simulink model "dieu_khien_canh_tay_may"  (R2023b)
settings: Solver=VariableStepAuto  StartTime=0.0  StopTime=3  RelTol=1e-3
values from neighbouring files (symbols this model uses):
  theta1_dot_init = 0    [tinh_toan_canh_tay_may.m]
  theta1_init = 0    [tinh_toan_canh_tay_may.m]
  theta2_dot_init = 0    [tinh_toan_canh_tay_may.m]
  theta2_init = 0    [tinh_toan_canh_tay_may.m]
settings Model: Creator=Admin  LastModifiedBy=Admin

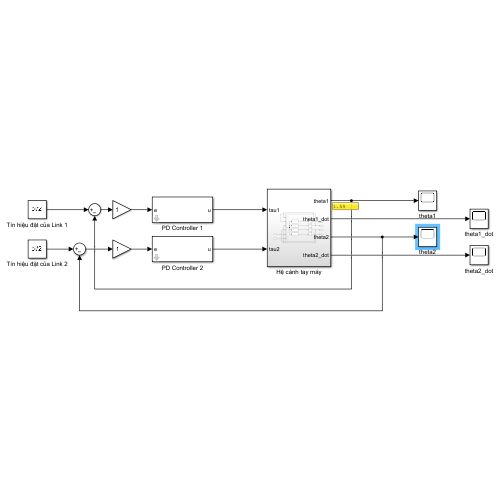
[thumbnail: Simulink's stored preview of the top-level diagram]
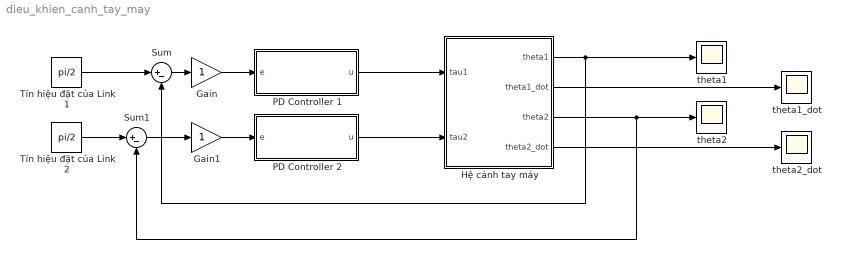
== system dieu_khien_canh_tay_may ==
  Gain : Gain
  Gain1 : Gain
  Hệ cánh tay máy : Subsystem
  PD Controller 1 : Subsystem  mask{Kp1=100, Kd1=20}
      mask prompts: Kp1 "Khâu Tỉ Lệ Kp1"; Kd1 "Khâu Vi Phân Kd1"
  PD Controller 2 : Subsystem  mask{Kp2=100, Kd2=20}
      mask prompts: Kp2 "Khâu Tỉ Lệ Kp2"; Kd2 "Khâu Vi Phân Kd2"
  Sum : Sum  Inputs=|+-
  Sum1 : Sum  Inputs=|+-
  Tín hiệu đặt của Link 1 : Constant  Value=pi/2
  Tín hiệu đặt của Link 2 : Constant  Value=pi/2
  theta1 : Scope
  theta1_dot : Scope
  theta2 : Scope
  theta2_dot : Scope
  wires:
  Hệ cánh tay máy/2(theta1_dot) -> theta1_dot/1
  Hệ cánh tay máy/3(theta2) -> theta2/1, Sum1/2
  Hệ cánh tay máy/4(theta2_dot) -> theta2_dot/1
  PD Controller 2/1(u) -> Hệ cánh tay máy/2(tau2)
  Tín hiệu đặt của Link 2/1 -> Sum1/1
  Tín hiệu đặt của Link 1/1 -> Sum/1
  Sum/1 -> Gain/1
  Sum1/1 -> Gain1/1
  Gain1/1 -> PD Controller 2/1(e)
  Hệ cánh tay máy/1(theta1) -> theta1/1, Sum/2
  Gain/1 -> PD Controller 1/1(e)
  PD Controller 1/1(u) -> Hệ cánh tay máy/1(tau1)

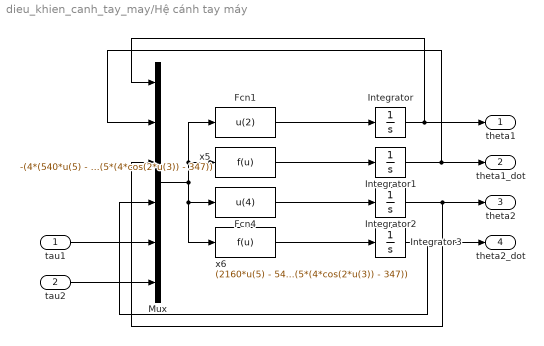
== system dieu_khien_canh_tay_may/Hệ cánh tay máy ==
  tau1 : Inport
  tau2 : Inport  Port=2
  Fcn1 : Fcn  Expr=u(2)
  Fcn4 : Fcn  Expr=u(4)
  Integrator : Integrator  InitialCondition=theta1_init
  Integrator1 : Integrator  InitialCondition=theta1_dot_init
  Integrator2 : Integrator  InitialCondition=theta2_init
  Integrator3 : Integrator  InitialCondition=theta2_dot_init
  Mux : Mux  Inputs=6
  x5 : Fcn  Expr=-(4*(540*u(5) - 540*u(6) + 98*cos(u(1) + 2*u(3)) - 3871*cos(u(1)) + 54*u(2)^2*sin(u(3)) + 54*u(4)^2*sin(u(3)) + 5*u(2)^2*sin(2*u(3)) - 100*u(6)*cos(u(3)) + 108*u(2)*u(4)*sin(u(3))))/(5*(4*cos(2*u(3)) - 347))
  x6 : Fcn  Expr=(2160*u(5) - 5410*u(6) - 1470*cos(u(1) - u(3)) + 392*cos(u(1) + 2*u(3)) + 4900*cos(u(1) + u(3)) - 15484*cos(u(1)) + 541*u(2)^2*sin(u(3)) + 216*u(4)^2*sin(u(3)) + 40*u(2)^2*sin(2*u(3)) + 20*u(4)^2*sin(2*u(3)) + 400*u(5)*cos(u(3)) - 800*u(6)*cos(u(3)) + 432*u(2)*u(4)*sin(u(3)) + 40*u(2)*u(4)*sin(2*u(3)))/(5*(4*cos(2*u(3)) - 347))
  theta1 : Outport
  theta1_dot : Outport  Port=2
  theta2 : Outport  Port=3
  theta2_dot : Outport  Port=4
  wires:
  tau2/1 -> Mux/6
  tau1/1 -> Mux/5
  Integrator1/1 -> Mux/2, theta1_dot/1
  Integrator/1 -> Mux/1, theta1/1
  Integrator2/1 -> Mux/3, theta2/1
  Integrator3/1 -> Mux/4, theta2_dot/1
  Fcn1/1 -> Integrator/1
  x5/1 -> Integrator1/1
  Fcn4/1 -> Integrator2/1
  x6/1 -> Integrator3/1
  Mux/1 -> Fcn1/1, x5/1, Fcn4/1, x6/1

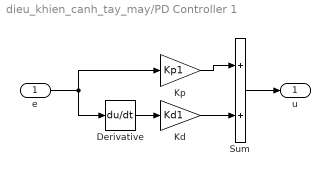
== system dieu_khien_canh_tay_may/PD Controller 1 ==
  e : Inport
  Derivative : Derivative
  Kd : Gain  Gain=Kd1
  Kp : Gain  Gain=Kp1
  Sum : Sum
  u : Outport
  wires:
  e/1 -> Derivative/1, Kp/1
  Derivative/1 -> Kd/1
  Kp/1 -> Sum/1
  Kd/1 -> Sum/2
  Sum/1 -> u/1

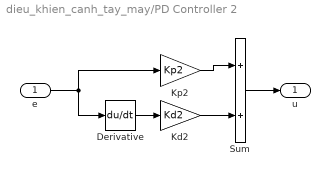
== system dieu_khien_canh_tay_may/PD Controller 2 ==
  e : Inport
  Derivative : Derivative
  Kd2 : Gain  Gain=Kd2
  Kp2 : Gain  Gain=Kp2
  Sum : Sum
  u : Outport
  wires:
  e/1 -> Derivative/1, Kp2/1
  Derivative/1 -> Kd2/1
  Kp2/1 -> Sum/1
  Kd2/1 -> Sum/2
  Sum/1 -> u/1
